simulink model "engine_core"  (R2026a)
settings: Solver=ode23t  StopTime=1039.5715
values from neighbouring files (symbols this model uses):
  Eng = struct()    [AeroDieselEngineParameters.m]
libraries: simulink x2
settings Model: Creator=asus  LastModifiedBy=asus

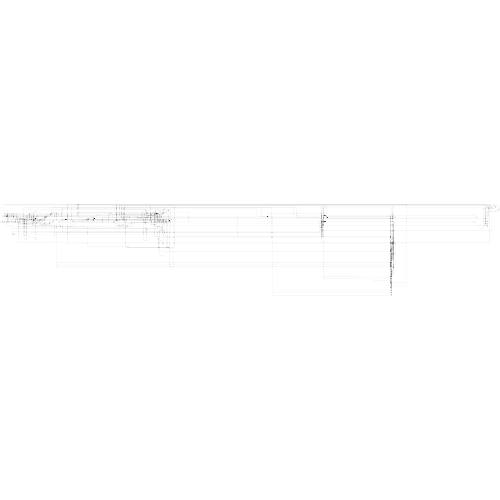
[thumbnail: Simulink's stored preview of the top-level diagram]
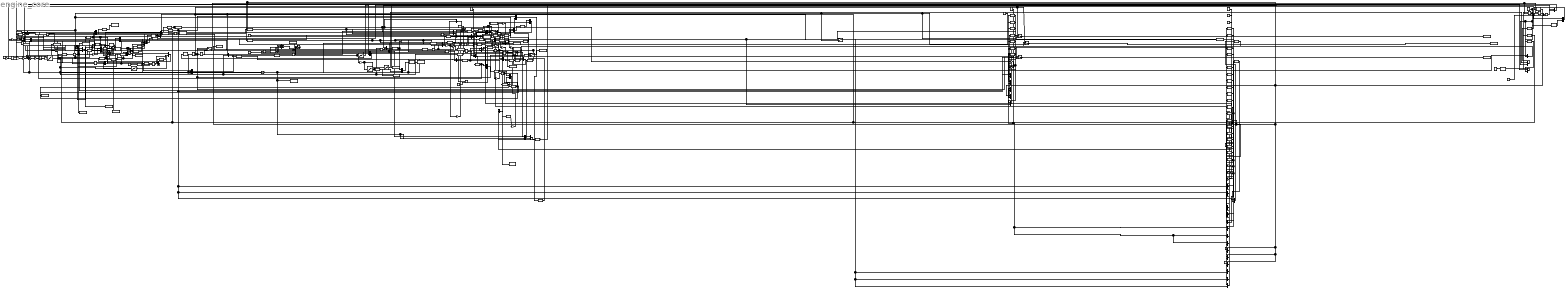
== system engine_core ==
  CmpEngineRunning : simulink/Logic and Bit Operations/Compare To Constant  relop=>  const=400  OutDataTypeStr=boolean
  ConstAlternatorHealth : Constant  Value=Eng.AlternatorHealth_init
  ConstAltitude : FromWorkspace  VariableName=MissionAltitude
  ConstBearingHealth : Constant  Value=Eng.BearingHealth_init
  ConstCoolingHealth : Constant  Value=Eng.CoolingHealth_init
  ConstDropoutNaNVibX : Constant  Value=NaN
  ConstElectricalLoad : Constant  Value=Eng.ElectricalLoad_kW
  ConstEpsilon : Constant  Value=1e-6
  ConstFuelDenomEps : Constant  Value=0.01
  ConstFueldelivHealth : Constant  Value=Eng.FuelDeliveryHealth_init
  ConstInjTimingDeg : Constant  Value=Eng.InjectionTimingDeg_init
  ConstInjhealthC1 : Constant  Value=Eng.InjectorHealth_c1_init
  ConstInjhealthC2 : Constant  Value=Eng.InjectorHealth_c2_init
  ConstInjhealthC3 : Constant  Value=Eng.InjectorHealth_c3_init
  ConstInjhealthC4 : Constant  Value=Eng.InjectorHealth_c4_init
  ConstIsatempoffset : FromWorkspace  VariableName=MissionIsaOffset
  ConstMdotEps : Constant  Value=0.001
  ConstMinrpmFloor : Constant  Value=400
  ConstOilpumpHealth : Constant  Value=Eng.OilPumpHealth_init
  ConstOne : Constant
  ConstPowerfloor : Constant  Value=0.001
  ConstSensorBiasC3 : Constant  Value=Eng.SensorBiasOffset_c3_degC
  ConstTurboEfficiencyDeg : Constant  Value=Eng.TurboEfficiencyDeg_init
  ConstZeroAfr : Constant  Value=0
  ConstZeroFuel : Constant  Value=0
  DivideFuelDeficitRatio : Product  Inputs=*/
  EnvService : ModelReference  ModelNameDialog=environment_service  SimulationMode=Normal  ModelReferenceVersion=1.2
  FcnActualPowerKw : Fcn  Expr=u[1]*(u[2]*2*pi/60)/1000
  FcnAfr : Fcn  Expr=u[1]/u[2]
  FcnAirmdot : Fcn  Expr=0.0017919*(u[1]/2/60)*(u[2]/(287.05*u[3]))
  FcnAlternatorPower : Fcn  Expr=u[1]*u[2]*Eng.AlternatorRatedPower_kW
  FcnBatteryCurrent : Fcn  Expr=u[1]*1000/u[2]
  FcnBatteryNetpower : Fcn  Expr=u[1]-u[2]
  FcnBatteryVoltage : Fcn  Expr=Eng.SystemVoltage_V*(0.85+0.15*u)
  FcnBoostBar : Fcn  Expr=(u[1]-u[2])/1e5
  FcnBsfcPenaltyFactor : Fcn  Expr=1+Eng.TimingDriftBSFCPenalty*u
  FcnCht1Net : Fcn  Expr=u[1]*1000-u[2]
  FcnCht1Reject : Fcn  Expr=Eng.CHTHeatTransferCoeff_W_per_K*(u[1]-u[2])
  FcnCht2Net : Fcn  Expr=u[1]*1000-u[2]
  FcnCht2Reject : Fcn  Expr=Eng.CHTHeatTransferCoeff_W_per_K*(u[1]-u[2])
  FcnCht3Net : Fcn  Expr=u[1]*1000-u[2]
  FcnCht3Reject : Fcn  Expr=Eng.CHTHeatTransferCoeff_W_per_K*(u[1]-u[2])
  FcnCht4Net : Fcn  Expr=u[1]*1000-u[2]
  FcnCht4Reject : Fcn  Expr=Eng.CHTHeatTransferCoeff_W_per_K*(u[1]-u[2])
  FcnEffectiveHeadroom : Fcn  Expr=1+(Eng.TurboAltitudeCompHeadroom-1)*(1-u)
  FcnEgtC1Raw : Fcn  Expr=u[1]+u[2]
  FcnEgtC2Raw : Fcn  Expr=u[1]+u[2]
  FcnEgtC3Raw : Fcn  Expr=u[1]+u[2]
  FcnEgtC4Raw : Fcn  Expr=u[1]+u[2]
  FcnEgtDegc : Fcn  Expr=u[1]+u[2]
  FcnEgtRise : Fcn  Expr=u[1]*1000/(Eng.CpExhaust_J_per_kgK*u[2])
  FcnEgtriseC{1..4} (4 alike) : Fcn  Expr=u[1]*1000/(Eng.CpExhaust_J_per_kgK*u[2])
  FcnExhaustfraction : Fcn  Expr=0.35+0*u[1]+Eng.TimingDriftExhaustPenalty*u[2]
  FcnExhaustmdot : Fcn  Expr=u[1]+u[2]
  FcnExhmdotC{1..4} (4 alike) : Fcn  Expr=u[1]+u[2]
  FcnFrictionScaled : Fcn  Expr=u[1]*(1+Eng.BearingFrictionGain*(1-u[2]))
  FcnFrictionpower : Fcn  Expr=u[1]*(u[2]*2*pi/60)
  FcnFuelFinal : Fcn  Expr=u[1]*u[2]
  FcnFuelFlow : Fcn  Expr=2.0+u[1]*u[2]/1000
  FcnFuelMdotKgs : Fcn  Expr=u/3600
  FcnFuelmdotC{1..4} (4 alike) : Fcn  Expr=u/3600
  FcnFuelpowerKw : Fcn  Expr=u*11.8889
  FcnFuelshareC{1..4} (4 alike) : Fcn  Expr=0.25*u[1]*u[2]
  FcnInjDurationMs : Fcn  Expr=u[1]/u[2]
  FcnInjFlowrate : Fcn  Expr=30*sqrt(u/1500)
  FcnInjQtyMg : Fcn  Expr=(u[1]*1e6/3600)/(4*(u[2]/2/60))
  FcnMapPa : Fcn  Expr=u[1]*u[2]
  FcnMapSealevelRef : Fcn  Expr=101325*u
  FcnMaxDeliverableFuel : Fcn  Expr=Eng.MaxRatedFuelFlow_kg_h*u
  FcnOilHeatTotal : Fcn  Expr=u[1]+u[2]
  FcnOilNet : Fcn  Expr=u[1]-u[2]
  FcnOilReject : Fcn  Expr=Eng.UAOilCooler_W_per_K*(u[1]-u[2])
  FcnOilpressure : Fcn  Expr=u[2]*(Eng.OilPressureIdle_bar+Eng.OilPumpGain_bar_per_rpm*(u[1]-Eng.IdleRPM_crank))
  FcnOilrejectScaled : Fcn  Expr=u[1]*u[2]
  FcnOtherlossesFraction : Fcn  Expr=1-u[1]-Eng.CoolantHeatFraction-u[2]
  FcnPambPa : Fcn  Expr=u*1000
  FcnPrActual : Fcn  Expr=1+u[1]*(u[2]-1)
  FcnPrCompensated : Fcn  Expr=u[1]*u[2]
  FcnPrFinalRef : Fcn  Expr=1+u[1]*(u[2]-1)
  FcnQOtherW : Fcn  Expr=u[1]*u[2]*1000
  FcnQexhaust : Fcn  Expr=u[1]*u[2]
  FcnQexhaustC{1..4} (4 alike) : Fcn  Expr=u[1]*u[2]
  FcnQtotalC{1..4} (4 alike) : Fcn  Expr=u*11.8889
  FcnRadiatorOut : Fcn  Expr=1330*(u[1]-u[2])
  FcnRadiatorScaled : Fcn  Expr=u[1]*u[2]
  FcnRatioNeeded : Fcn  Expr=101325/u
  FcnRefPowerKw : Fcn  Expr=u[1]*(u[2]*2*pi/60)/1000
  FcnRpmFraction : Fcn  Expr=u/Eng.RatedRPM_crank
  FcnRpmRatioSq : Fcn  Expr=(u/Eng.RatedRPM_crank)^2
  FcnTambK : Fcn  Expr=u+273.15
  FcnTcompoutK : Fcn  Expr=u[1]*(1+(u[2]^0.285714-1)/0.7)
  FcnTimingActual : Fcn  Expr=u[1]-Eng.InjectionTimingDriftMax_deg*u[2]
  FcnTintakeDegc : Fcn  Expr=u-273.15
  FcnTintakeK : Fcn  Expr=u[1]-0.75*(u[1]-u[2])
  FcnTorqueFinal : Fcn  Expr=u[1]*u[2]
  FcnTorqueFinal2 : Fcn  Expr=u[1]*u[2]
  FcnTorquePenaltyFactor : Fcn  Expr=1-Eng.TimingDriftTorquePenalty*u
  FcnTorqueScaleFactor : Fcn  Expr=u[1]/u[2]
  FcnTorqueScaledV2 : Fcn  Expr=u[1]*u[2]
  FcnVibrationOrder1x : Fcn  Expr=Eng.VibrationImbalanceGain_g*(1-u[2])*u[1]
  FcnVibrationRmsX : Fcn  Expr=sqrt(Eng.VibrationBaseline_g^2+u^2)
  FcnWorkfraction : Fcn  Expr=u[1]/u[2]
  GainAirmdotPercyl : Gain  Gain=0.25
  GainCht1Rate : Gain  Gain=1/Eng.CHTThermalMass_J_per_K
  GainCht2Rate : Gain  Gain=1/Eng.CHTThermalMass_J_per_K
  GainCht3Rate : Gain  Gain=1/Eng.CHTThermalMass_J_per_K
  GainCht4Rate : Gain  Gain=1/Eng.CHTThermalMass_J_per_K
  GainCoolantRate : Gain  Gain=1/Eng.CoolantThermalMass_J_per_K
  GainFriction : Gain  Gain=Eng.FrictionCoeff_Nm_per_rpm
  GainGearboxReflect : Gain  Gain=1/Eng.GearboxReductionRatio
  GainGearboxToProp : Gain  Gain=1/Eng.GearboxReductionRatio
  GainInvinertia : Gain  Gain=1/Eng.CrankInertia_kgm2
  GainLambda : Gain  Gain=1/Eng.StoichAFR_diesel
  GainLoadfraction : Gain  Gain=1/123.5
  GainMapKpa : Gain  Gain=0.001
  GainOilRate : Gain  Gain=1/Eng.OilThermalMass_J_per_K
  GainProploadcoeff : Gain  Gain=Eng.PropLoadCoeff_Nm_per_prop_rpm2
  GainQcoolant : Gain  Gain=Eng.CoolantHeatFraction
  GainQcoolantDirect : Gain  Gain=1000*(1-Eng.HeadHeatShareOfCoolant)
  GainQhead : Gain  Gain=Eng.HeadHeatShareOfCoolant
  GainQheadC{1..4} (4 alike) : Gain  Gain=Eng.CoolantHeatFraction*Eng.HeadHeatShareOfCoolant
  GainRadstorpm : Gain  Gain=60/(2*pi)
  GainSocRate : Gain  Gain=1000/(Eng.BatteryCapacity_Ah*3600*Eng.SystemVoltage_V)
  GainVibrationRmsZ : Gain  Gain=0.3
  IntChtC{1..4} (4 alike) : Integrator  InitialCondition=Eng.CHTInit_degC
  IntCoolant : Integrator  InitialCondition=Eng.CoolantTempInit_degC
  IntOil : Integrator  InitialCondition=Eng.OilTempInit_degC
  IntSoc : Integrator  InitialCondition=0.8  LimitOutput=on  UpperSaturationLimit=1  LowerSaturationLimit=0
  Integrator : Integrator  InitialCondition=Eng.IdleRPM_crank*2*pi/60
  LutBsfc : Lookup_n-D  NumberOfTableDimensions=1  BreakpointsForDimension1=Eng.BSFCMap.RefPower_kW  Table=Eng.BSFCMap.BSFC_g_per_kWh  ExtrapMethod=Clip  InternalRulePriority=Speed  RndMeth=Simplest
  LutInjTiming : Lookup_n-D  NumberOfTableDimensions=1  BreakpointsForDimension1=Eng.InjectionTimingMap.LoadFraction  Table=Eng.InjectionTimingMap.Timing_degBTDC  ExtrapMethod=Clip  InternalRulePriority=Speed  RndMeth=Simplest
  LutPrFull : Lookup_n-D  NumberOfTableDimensions=1  BreakpointsForDimension1=Eng.TurboBoostMap.RPM_crank  Table=Eng.TurboBoostMap.PressureRatio  ExtrapMethod=Clip  InternalRulePriority=Speed  RndMeth=Simplest
  LutRailPressure : Lookup_n-D  NumberOfTableDimensions=1  BreakpointsForDimension1=Eng.RailPressureMap.LoadFraction  Table=Eng.RailPressureMap.Pressure_bar  ExtrapMethod=Clip  InternalRulePriority=Speed  RndMeth=Simplest
  LutTorquecurve : Lookup_n-D  NumberOfTableDimensions=1  BreakpointsForDimension1=Eng.TorqueCurve.RPM_crank  Table=Eng.TorqueCurve.Torque_Nm  ExtrapMethod=Clip  InternalRulePriority=Speed  RndMeth=Simplest
  MathRpmsquared : Math  Operator=square  SignedPower=on  RndMeth=Zero
  MemoryStuckC3 : Memory
  MinmaxCompfactor : MinMax  Inputs=2
  MinmaxExhmdotFloor : MinMax  Function=max  Inputs=2
  MinmaxFuelActual : MinMax  Inputs=2
  MinmaxFuelDenomFloor : MinMax  Function=max  Inputs=2
  MinmaxFuelmdotFloor : MinMax  Function=max  Inputs=2
  MinmaxFuelpowerFloor : MinMax  Function=max  Inputs=2
  MinmaxRpmFloor : MinMax  Function=max  Inputs=2
  MinmaxRpmfracCap : MinMax  Inputs=2
  MuxActualpwrFuelpwr : Mux  Inputs=2
  MuxAirFuel : Mux  Inputs=2
  MuxAirFuelMdot : Mux  Inputs=2
  MuxBatteryNetpower : Mux  Inputs=2
  MuxCapfracHealth : Mux  Inputs=2
  MuxCht1Coolant : Mux  Inputs=2
  MuxCht1Net : Mux  Inputs=2
  MuxCht2Coolant : Mux  Inputs=2
  MuxCht2Net : Mux  Inputs=2
  MuxCht3Coolant : Mux  Inputs=2
  MuxCht3Net : Mux  Inputs=2
  MuxCht4Coolant : Mux  Inputs=2
  MuxCht4Net : Mux  Inputs=2
  MuxCoolantAmbient : Mux  Inputs=2
  MuxEgtC{1..4} (4 alike) : Mux  Inputs=2
  MuxEgtriseC{1..4} (4 alike) : Mux  Inputs=2
  MuxExhfracTimingdeg : Mux  Inputs=2
  MuxExhmdotC{1..4} (4 alike) : Mux  Inputs=2
  MuxFrictionHealth : Mux  Inputs=2
  MuxFrictionOther : Mux  Inputs=2
  MuxFrictionpower : Mux  Inputs=2
  MuxFuelHealthC{1..4} (4 alike) : Mux  Inputs=2
  MuxFuelTimingpenalty : Mux  Inputs=2
  MuxFuelflowRpm : Mux  Inputs=2
  MuxFuelpowerOtherfrac : Mux  Inputs=2
  MuxFuelpwrExhfrac : Mux  Inputs=2
  MuxImbalance : Mux  Inputs=2
  MuxMapActualRef : Mux  Inputs=2
  MuxMapPambBoost : Mux  Inputs=2
  MuxOilCoolant : Mux  Inputs=2
  MuxOilNet : Mux  Inputs=2
  MuxOilcoolerHealth : Mux  Inputs=2
  MuxOtherlosses : Mux  Inputs=2
  MuxPambPr : Mux  Inputs=2
  MuxPowerVoltage : Mux  Inputs=2
  MuxPrrawCompfactor : Mux  Inputs=2
  MuxQexhC{1..4} (4 alike) : Mux  Inputs=2
  MuxQexhMdot : Mux  Inputs=2
  MuxQtyFlowrate : Mux  Inputs=2
  MuxRadiatorHealth : Mux  Inputs=2
  MuxRefpwrBsfc : Mux  Inputs=2
  MuxRpmMapTintake : Mux  Inputs=3
  MuxRpmOilhealth : Mux  Inputs=2
  MuxTambPr : Mux  Inputs=2
  MuxTcompoutTamb : Mux  Inputs=2
  MuxThrPrfull : Mux  Inputs=2
  MuxThrPrrawRef : Mux  Inputs=2
  MuxTimingDrift : Mux  Inputs=2
  MuxTintakeEgtrise : Mux  Inputs=2
  MuxTorqueFueldeficit : Mux  Inputs=2
  MuxTorqueScale : Mux  Inputs=2
  MuxTorqueTimingpenalty : Mux  Inputs=2
  MuxTrqRpmActualpwr : Mux  Inputs=2
  MuxTrqRpmRefpwr : Mux  Inputs=2
  ProdEnginetorque : Product
  RampSensordriftC3 : simulink/Sources/Ramp  slope=Eng.SensorDriftRate_c3_degC_per_s  start=0  InitialOutput=0
  RandnSensorNoiseC3 : RandomNumber  Variance=Eng.SensorNoiseSigma_c3_degC^2  Seed=42  SampleTime=0.1
  ScopeRpm : Scope
  ScopeTorque : Scope
  StepDropoutOffVibX : Step  Time=Eng.SensorDropoutEndTime_s  SampleTime=0
  StepDropoutOnVibX : Step  Time=Eng.SensorDropoutStartTime_s  SampleTime=0
  StepStuckActiveC3 : Step  Time=Eng.SensorStuckActivationTime_s  SampleTime=0
  StepThrottle : FromWorkspace  VariableName=MissionThrottle
  SumCht3Reported : Sum  Inputs=++++
  SumChtRejects : Sum  Inputs=++++
  SumCoolantHeatin : Sum  Inputs=+++
  SumCoolantNet : Sum  Inputs=+-
  SumDropoutControlVibX : Sum  Inputs=+-
  SumNettorque : Sum  Inputs=+--
  SwitchAfrGate : Switch  Criteria=u2 > Threshold  Threshold=0.5  SaturateOnIntegerOverflow=off  InputSameDT=off
  SwitchDropoutVibX : Switch  Criteria=u2 > Threshold  Threshold=0.5  SaturateOnIntegerOverflow=off  InputSameDT=off
  SwitchEgtC1Gate : Switch  Criteria=u2 > Threshold  Threshold=0.5  SaturateOnIntegerOverflow=off  InputSameDT=off
  SwitchEgtC2Gate : Switch  Criteria=u2 > Threshold  Threshold=0.5  SaturateOnIntegerOverflow=off  InputSameDT=off
  SwitchEgtC3Gate : Switch  Criteria=u2 > Threshold  Threshold=0.5  SaturateOnIntegerOverflow=off  InputSameDT=off
  SwitchEgtC4Gate : Switch  Criteria=u2 > Threshold  Threshold=0.5  SaturateOnIntegerOverflow=off  InputSameDT=off
  SwitchEgtGate : Switch  Criteria=u2 > Threshold  Threshold=0.5  SaturateOnIntegerOverflow=off  InputSameDT=off
  SwitchFuelGate : Switch  Criteria=u2 > Threshold  Threshold=0.5  SaturateOnIntegerOverflow=off  InputSameDT=off
  SwitchStuckC3 : Switch  Criteria=u2 > Threshold  Threshold=0.5  SaturateOnIntegerOverflow=off  InputSameDT=off
  TowsAfr : ToWorkspace  VariableName=afr_out  SaveFormat=Timeseries  SampleTime=-1
  TowsAirmdot : ToWorkspace  VariableName=air_mdot_out  SaveFormat=Timeseries  SampleTime=-1
  TowsAltpower : ToWorkspace  VariableName=alt_power_out  SaveFormat=Timeseries  SampleTime=-1
  TowsAmbientTemp : ToWorkspace  VariableName=ambient_temp_out  SaveFormat=Timeseries  SampleTime=-1
  TowsBattcurrent : ToWorkspace  VariableName=batt_current_out  SaveFormat=Timeseries  SampleTime=-1
  TowsBattvoltage : ToWorkspace  VariableName=batt_voltage_out  SaveFormat=Timeseries  SampleTime=-1
  TowsBoost : ToWorkspace  VariableName=boost_pressure_out  SaveFormat=Timeseries  SampleTime=-1
  TowsCht1 : ToWorkspace  VariableName=cht1_out  SaveFormat=Timeseries  SampleTime=-1
  TowsCht2 : ToWorkspace  VariableName=cht2_out  SaveFormat=Timeseries  SampleTime=-1
  TowsCht3 : ToWorkspace  VariableName=cht3_out  SaveFormat=Timeseries  SampleTime=-1
  TowsCht3Reported : ToWorkspace  VariableName=cht3_reported_out  SaveFormat=Timeseries  SampleTime=-1
  TowsCht4 : ToWorkspace  VariableName=cht4_out  SaveFormat=Timeseries  SampleTime=-1
  TowsCoolant : ToWorkspace  VariableName=coolant_out  SaveFormat=Timeseries  SampleTime=-1
  TowsDensity : ToWorkspace  VariableName=air_density_out  SaveFormat=Timeseries  SampleTime=-1
  TowsEgt : ToWorkspace  VariableName=egt_out  SaveFormat=Timeseries  SampleTime=-1
  TowsEgtC1 : ToWorkspace  VariableName=egt_c1_out  SaveFormat=Timeseries  SampleTime=-1
  TowsEgtC2 : ToWorkspace  VariableName=egt_c2_out  SaveFormat=Timeseries  SampleTime=-1
  TowsEgtC3 : ToWorkspace  VariableName=egt_c3_out  SaveFormat=Timeseries  SampleTime=-1
  TowsEgtC4 : ToWorkspace  VariableName=egt_c4_out  SaveFormat=Timeseries  SampleTime=-1
  TowsFuelflow : ToWorkspace  VariableName=fuel_flow_out  SaveFormat=Timeseries  SampleTime=-1
  TowsInjduration : ToWorkspace  VariableName=inj_duration_out  SaveFormat=Timeseries  SampleTime=-1
  TowsInjqty : ToWorkspace  VariableName=inj_qty_out  SaveFormat=Timeseries  SampleTime=-1
  TowsInjtiming : ToWorkspace  VariableName=inj_timing_out  SaveFormat=Timeseries  SampleTime=-1
  TowsLambda : ToWorkspace  VariableName=lambda_out  SaveFormat=Timeseries  SampleTime=-1
  TowsMap : ToWorkspace  VariableName=map_out  SaveFormat=Timeseries  SampleTime=-1
  TowsOil : ToWorkspace  VariableName=oil_out  SaveFormat=Timeseries  SampleTime=-1
  TowsOilpressure : ToWorkspace  VariableName=oil_pressure_out  SaveFormat=Timeseries  SampleTime=-1
  TowsPressure : ToWorkspace  VariableName=ambient_pressure_out  SaveFormat=Timeseries  SampleTime=-1
  TowsQhead : ToWorkspace  VariableName=q_head_out  SaveFormat=Timeseries  SampleTime=-1
  TowsQtotal : ToWorkspace  VariableName=q_total_out  SaveFormat=Timeseries  SampleTime=-1
  TowsRailpressure : ToWorkspace  VariableName=rail_pressure_out  SaveFormat=Timeseries  SampleTime=-1
  TowsRpm : ToWorkspace  VariableName=rpm_out  SaveFormat=Timeseries  SampleTime=-1
  TowsSoc : ToWorkspace  VariableName=soc_out  SaveFormat=Timeseries  SampleTime=-1
  TowsTintake : ToWorkspace  VariableName=intake_temp_out  SaveFormat=Timeseries  SampleTime=-1
  TowsTorque : ToWorkspace  VariableName=torque_out  SaveFormat=Timeseries  SampleTime=-1
  TowsVibOrder1x : ToWorkspace  VariableName=vib_order1x_out  SaveFormat=Timeseries  SampleTime=-1
  TowsVibRmsX : ToWorkspace  VariableName=vib_rms_x_out  SaveFormat=Timeseries  SampleTime=-1
  TowsVibRmsZ : ToWorkspace  VariableName=vib_rms_z_out  SaveFormat=Timeseries  SampleTime=-1
  wires:
  Integrator/1 -> GainRadstorpm/1
  GainInvinertia/1 -> Integrator/1
  GainGearboxReflect/1 -> SumNettorque/2
  GainGearboxToProp/1 -> MathRpmsquared/1
  GainProploadcoeff/1 -> GainGearboxReflect/1
  MathRpmsquared/1 -> GainProploadcoeff/1
  SumNettorque/1 -> GainInvinertia/1
  FcnTambK/1 -> MuxTcompoutTamb/2, MuxTambPr/1
  MuxPambPr/1 -> FcnMapPa/1
  FcnPrActual/1 -> MuxTambPr/2, MuxPambPr/2
  FcnBoostBar/1 -> TowsBoost/1
  MuxMapPambBoost/1 -> FcnBoostBar/1
  MuxRpmMapTintake/1 -> FcnAirmdot/1
  MuxTorqueScale/1 -> FcnTorqueScaledV2/1
  FcnTorqueScaleFactor/1 -> MuxTorqueScale/2
  MuxMapActualRef/1 -> FcnTorqueScaleFactor/1
  FcnMapSealevelRef/1 -> MuxMapActualRef/2
  FcnPrFinalRef/1 -> FcnMapSealevelRef/1
  MuxThrPrrawRef/1 -> FcnPrFinalRef/1
  FcnPrCompensated/1 -> MuxThrPrfull/2
  FcnMapPa/1 -> MuxMapActualRef/1, MuxRpmMapTintake/2, GainMapKpa/1, MuxMapPambBoost/1
  MuxThrPrfull/1 -> FcnPrActual/1
  MuxTambPr/1 -> FcnTcompoutK/1
  FcnTcompoutK/1 -> MuxTcompoutTamb/1
  MuxTcompoutTamb/1 -> FcnTintakeK/1
  LutBsfc/1 -> MuxRefpwrBsfc/2
  FcnRefPowerKw/1 -> GainLoadfraction/1, MuxRefpwrBsfc/1, LutBsfc/1
  MuxTrqRpmRefpwr/1 -> FcnRefPowerKw/1
  ProdEnginetorque/1 -> MuxTrqRpmRefpwr/1, MuxTorqueScale/1
  FcnInjDurationMs/1 -> TowsInjduration/1
  LutInjTiming/1 -> MuxTimingDrift/1
  GainLoadfraction/1 -> LutRailPressure/1, LutInjTiming/1
  LutRailPressure/1 -> TowsRailpressure/1, FcnInjFlowrate/1
  FcnInjQtyMg/1 -> TowsInjqty/1, MuxQtyFlowrate/1
  FcnInjFlowrate/1 -> MuxQtyFlowrate/2
  MuxQtyFlowrate/1 -> FcnInjDurationMs/1
  FcnTintakeK/1 -> FcnTintakeDegc/1, MuxRpmMapTintake/3
  GainMapKpa/1 -> TowsMap/1
  MinmaxRpmFloor/1 -> MuxFuelflowRpm/2
  ConstMinrpmFloor/1 -> MinmaxRpmFloor/2
  MuxFuelflowRpm/1 -> FcnInjQtyMg/1
  ConstZeroFuel/1 -> SwitchFuelGate/3
  FcnFuelFlow/1 -> SwitchFuelGate/1
  MuxRefpwrBsfc/1 -> FcnFuelFlow/1
  MuxActualpwrFuelpwr/1 -> FcnWorkfraction/1
  MinmaxFuelpowerFloor/1 -> MuxActualpwrFuelpwr/2
  FcnActualPowerKw/1 -> MuxActualpwrFuelpwr/1
  MuxTrqRpmActualpwr/1 -> FcnActualPowerKw/1
  ConstPowerfloor/1 -> MinmaxFuelpowerFloor/2
  ConstMdotEps/1 -> MinmaxExhmdotFloor/2
  SwitchEgtGate/1 -> TowsEgt/1
  MinmaxExhmdotFloor/1 -> MuxQexhMdot/2
  MuxFuelpwrExhfrac/1 -> FcnQexhaust/1
  FcnQexhaust/1 -> MuxQexhMdot/1
  GainOilRate/1 -> IntOil/1
  FcnOilNet/1 -> GainOilRate/1
  GainCoolantRate/1 -> IntCoolant/1
  MuxCht1Coolant/1 -> FcnCht1Reject/1
  FcnCht2Reject/1 -> SumChtRejects/2, MuxCht2Net/2
  GainCht2Rate/1 -> IntChtC2/1
  FcnAirmdot/1 -> GainAirmdotPercyl/1, MuxAirFuel/1, MuxAirFuelMdot/1, TowsAirmdot/1
  SwitchAfrGate/1 -> GainLambda/1, TowsAfr/1
  FcnAfr/1 -> SwitchAfrGate/1
  MuxAirFuel/1 -> FcnAfr/1
  FcnEgtRise/1 -> MuxTintakeEgtrise/2
  MuxQexhMdot/1 -> FcnEgtRise/1
  MuxOilcoolerHealth/1 -> FcnOilrejectScaled/1
  ConstOilpumpHealth/1 -> MuxRpmOilhealth/2, MuxOilcoolerHealth/2
  FcnRadiatorScaled/1 -> SumCoolantNet/2
  MuxRadiatorHealth/1 -> FcnRadiatorScaled/1
  ConstCoolingHealth/1 -> MuxRadiatorHealth/2
  SumCoolantHeatin/1 -> SumCoolantNet/1
  FcnOilReject/1 -> MuxOilcoolerHealth/1
  SumChtRejects/1 -> SumCoolantHeatin/1
  ConstZeroAfr/1 -> SwitchAfrGate/3
  MuxAirFuelMdot/1 -> FcnExhaustmdot/1
  FcnFuelMdotKgs/1 -> MuxAirFuelMdot/2, MinmaxFuelmdotFloor/1
  MuxCht1Net/1 -> FcnCht1Net/1
  FcnCht1Reject/1 -> MuxCht1Net/2, SumChtRejects/1
  MuxCoolantAmbient/1 -> FcnRadiatorOut/1
  FcnRadiatorOut/1 -> MuxRadiatorHealth/1
  SumCoolantNet/1 -> GainCoolantRate/1
  FcnExhaustmdot/1 -> MinmaxExhmdotFloor/1
  ConstEpsilon/1 -> MinmaxFuelmdotFloor/2
  MinmaxFuelmdotFloor/1 -> MuxAirFuel/2
  LutTorquecurve/1 -> ProdEnginetorque/2
  FcnOilpressure/1 -> TowsOilpressure/1
  MuxOilCoolant/1 -> FcnOilReject/1
  MuxRpmOilhealth/1 -> FcnOilpressure/1
  IntChtC2/1 -> TowsCht2/1, MuxCht2Coolant/1
  FcnCht3Net/1 -> GainCht3Rate/1
  MuxCht3Net/1 -> FcnCht3Net/1
  FcnCht3Reject/1 -> MuxCht3Net/2, SumChtRejects/3
  FcnCht2Net/1 -> GainCht2Rate/1
  MuxCht2Net/1 -> FcnCht2Net/1
  MuxCht2Coolant/1 -> FcnCht2Reject/1
  GainCht1Rate/1 -> IntChtC1/1
  FcnCht1Net/1 -> GainCht1Rate/1
  IntOil/1 -> MuxOilCoolant/1, TowsOil/1
  MuxPowerVoltage/1 -> FcnBatteryCurrent/1
  GainSocRate/1 -> IntSoc/1
  FcnBatteryNetpower/1 -> MuxPowerVoltage/1, GainSocRate/1
  MuxBatteryNetpower/1 -> FcnBatteryNetpower/1
  ConstElectricalLoad/1 -> MuxBatteryNetpower/2
  MuxCapfracHealth/1 -> FcnAlternatorPower/1
  ConstAlternatorHealth/1 -> MuxCapfracHealth/2
  MinmaxRpmfracCap/1 -> MuxCapfracHealth/1
  ConstOne/1 -> MinmaxRpmfracCap/2
  FcnRpmFraction/1 -> MinmaxRpmfracCap/1
  MuxCht3Coolant/1 -> FcnCht3Reject/1
  MuxCht4Net/1 -> FcnCht4Net/1
  FcnCht4Net/1 -> GainCht4Rate/1
  GainCht4Rate/1 -> IntChtC4/1
  GainQhead/1 -> TowsQhead/1
  GainQcoolantDirect/1 -> SumCoolantHeatin/3
  GainQcoolant/1 -> GainQcoolantDirect/1, GainQhead/1
  IntChtC1/1 -> MuxCht1Coolant/1, TowsCht1/1
  FcnOilHeatTotal/1 -> MuxOilNet/1
  MuxFrictionOther/1 -> FcnOilHeatTotal/1
  FcnQOtherW/1 -> MuxFrictionOther/2
  MuxOilNet/1 -> FcnOilNet/1
  FcnFrictionpower/1 -> MuxFrictionOther/1
  GainLambda/1 -> TowsLambda/1
  FcnOilrejectScaled/1 -> SumCoolantHeatin/2, MuxOilNet/2
  ConstInjhealthC1/1 -> MuxFuelHealthC1/2
  MuxFuelHealthC1/1 -> FcnFuelshareC1/1
  FcnFuelshareC1/1 -> FcnFuelmdotC1/1, FcnQtotalC1/1
  FcnQtotalC1/1 -> MuxQexhC1/1, GainQheadC1/1
  GainQheadC1/1 -> MuxCht1Net/1
  MuxQexhC1/1 -> FcnQexhaustC1/1
  GainAirmdotPercyl/1 -> MuxExhmdotC4/1, MuxExhmdotC3/1, MuxExhmdotC2/1, MuxExhmdotC1/1
  FcnFuelmdotC1/1 -> MuxExhmdotC1/2
  MuxExhmdotC1/1 -> FcnExhmdotC1/1
  FcnQexhaustC1/1 -> MuxEgtriseC1/1
  FcnExhmdotC1/1 -> MuxEgtriseC1/2
  MuxEgtriseC1/1 -> FcnEgtriseC1/1
  FcnEgtriseC1/1 -> MuxEgtC1/2
  MuxEgtC1/1 -> FcnEgtC1Raw/1
  SwitchEgtC1Gate/1 -> TowsEgtC1/1
  FcnEgtC1Raw/1 -> SwitchEgtC1Gate/1
  ConstInjhealthC2/1 -> MuxFuelHealthC2/2
  MuxFuelHealthC2/1 -> FcnFuelshareC2/1
  FcnFuelshareC2/1 -> FcnQtotalC2/1, FcnFuelmdotC2/1
  FcnQtotalC2/1 -> MuxQexhC2/1, GainQheadC2/1
  GainQheadC2/1 -> MuxCht2Net/1
  MuxQexhC2/1 -> FcnQexhaustC2/1
  FcnFuelmdotC2/1 -> MuxExhmdotC2/2
  MuxExhmdotC2/1 -> FcnExhmdotC2/1
  FcnQexhaustC2/1 -> MuxEgtriseC2/1
  FcnExhmdotC2/1 -> MuxEgtriseC2/2
  MuxEgtriseC2/1 -> FcnEgtriseC2/1
  FcnEgtriseC2/1 -> MuxEgtC2/2
  MuxEgtC2/1 -> FcnEgtC2Raw/1
  ConstInjhealthC3/1 -> MuxFuelHealthC3/2
  MuxFuelHealthC3/1 -> FcnFuelshareC3/1
  FcnFuelshareC3/1 -> FcnQtotalC3/1, FcnFuelmdotC3/1
  FcnQtotalC3/1 -> MuxQexhC3/1, GainQheadC3/1
  GainQheadC3/1 -> MuxCht3Net/1
  MuxQexhC3/1 -> FcnQexhaustC3/1
  FcnFuelmdotC3/1 -> MuxExhmdotC3/2
  MuxExhmdotC3/1 -> FcnExhmdotC3/1
  FcnQexhaustC3/1 -> MuxEgtriseC3/1
  FcnExhmdotC3/1 -> MuxEgtriseC3/2
  MuxEgtriseC3/1 -> FcnEgtriseC3/1
  FcnEgtriseC3/1 -> MuxEgtC3/2
  MuxEgtC3/1 -> FcnEgtC3Raw/1
  ConstInjhealthC4/1 -> MuxFuelHealthC4/2
  MuxFuelHealthC4/1 -> FcnFuelshareC4/1
  FcnFuelshareC4/1 -> FcnQtotalC4/1, FcnFuelmdotC4/1
  FcnQtotalC4/1 -> MuxQexhC4/1, GainQheadC4/1
  GainQheadC4/1 -> MuxCht4Net/1
  MuxQexhC4/1 -> FcnQexhaustC4/1
  FcnFuelmdotC4/1 -> MuxExhmdotC4/2
  MuxExhmdotC4/1 -> FcnExhmdotC4/1
  FcnQexhaustC4/1 -> MuxEgtriseC4/1
  FcnExhmdotC4/1 -> MuxEgtriseC4/2
  SwitchEgtC3Gate/1 -> TowsEgtC3/1
  SwitchEgtC2Gate/1 -> TowsEgtC2/1
  FcnEgtC3Raw/1 -> SwitchEgtC3Gate/1
  FcnEgtC2Raw/1 -> SwitchEgtC2Gate/1
  FcnEffectiveHeadroom/1 -> MinmaxCompfactor/2
  ConstTurboEfficiencyDeg/1 -> FcnEffectiveHeadroom/1
  FcnFuelpowerKw/1 -> MuxFuelpowerOtherfrac/1, MuxFuelpwrExhfrac/1, MinmaxFuelpowerFloor/1, GainQcoolant/1, TowsQtotal/1
  FcnOtherlossesFraction/1 -> MuxFuelpowerOtherfrac/2
  MuxFuelpowerOtherfrac/1 -> FcnQOtherW/1
  IntChtC4/1 -> MuxCht4Coolant/1, TowsCht4/1
  FcnCht4Reject/1 -> SumChtRejects/4, MuxCht4Net/2
  MuxCht4Coolant/1 -> FcnCht4Reject/1
  IntCoolant/1 -> MuxOilCoolant/2, MuxCoolantAmbient/1, MuxCht3Coolant/2, MuxCht4Coolant/2, TowsCoolant/1, MuxCht2Coolant/2, MuxCht1Coolant/2
  FcnAlternatorPower/1 -> TowsAltpower/1, MuxBatteryNetpower/1
  MuxPrrawCompfactor/1 -> FcnPrCompensated/1
  FcnPambPa/1 -> FcnRatioNeeded/1, MuxPambPr/1, MuxMapPambBoost/2
  LutPrFull/1 -> MuxPrrawCompfactor/1, MuxThrPrrawRef/2
  FcnRatioNeeded/1 -> MinmaxCompfactor/1
  MinmaxCompfactor/1 -> MuxPrrawCompfactor/2
  RampSensordriftC3/1 -> SumCht3Reported/2
  IntChtC3/1 -> MuxCht3Coolant/1, TowsCht3/1, SumCht3Reported/1
  GainCht3Rate/1 -> IntChtC3/1
  FcnRpmRatioSq/1 -> MuxImbalance/1
  FcnFrictionScaled/1 -> MuxFrictionpower/1, SumNettorque/3
  MuxFrictionHealth/1 -> FcnFrictionScaled/1
  ConstBearingHealth/1 -> MuxImbalance/2, MuxFrictionHealth/2
  MuxFrictionpower/1 -> FcnFrictionpower/1
  GainRadstorpm/1 -> MuxRpmMapTintake/1, MinmaxRpmFloor/1, FcnRpmFraction/1, MuxTrqRpmActualpwr/2, MuxRpmOilhealth/1, MuxTrqRpmRefpwr/2, CmpEngineRunning/1, LutPrFull/1, GainFriction/1, MuxFrictionpower/2, FcnRpmRatioSq/1, TowsRpm/1, ScopeRpm/1, GainGearboxToProp/1, LutTorquecurve/1
  GainFriction/1 -> MuxFrictionHealth/1
  GainVibrationRmsZ/1 -> TowsVibRmsZ/1
  MuxImbalance/1 -> FcnVibrationOrder1x/1
  EnvService/1 -> FcnPambPa/1, TowsPressure/1
  EnvService/3 -> TowsDensity/1
  EnvService/2 -> SwitchEgtC2Gate/3, FcnTambK/1, SwitchEgtC3Gate/3, SwitchEgtC4Gate/3, SwitchEgtC1Gate/3, SwitchEgtGate/3, MuxCoolantAmbient/2, TowsAmbientTemp/1
  FcnVibrationRmsX/1 -> GainVibrationRmsZ/1, SwitchDropoutVibX/3
  FcnVibrationOrder1x/1 -> FcnVibrationRmsX/1, TowsVibOrder1x/1
  FcnBatteryVoltage/1 -> TowsBattvoltage/1, MuxPowerVoltage/2
  IntSoc/1 -> TowsSoc/1, FcnBatteryVoltage/1
  FcnEgtDegc/1 -> SwitchEgtGate/1
  MuxTintakeEgtrise/1 -> FcnEgtDegc/1
  FcnBatteryCurrent/1 -> TowsBattcurrent/1
  CmpEngineRunning/1 -> SwitchEgtGate/2, SwitchEgtC2Gate/2, SwitchAfrGate/2, SwitchFuelGate/2, SwitchEgtC3Gate/2, SwitchEgtC4Gate/2, SwitchEgtC1Gate/2
  FcnEgtC4Raw/1 -> SwitchEgtC4Gate/1
  SwitchEgtC4Gate/1 -> TowsEgtC4/1
  MuxEgtC4/1 -> FcnEgtC4Raw/1
  FcnEgtriseC4/1 -> MuxEgtC4/2
  MuxEgtriseC4/1 -> FcnEgtriseC4/1
  FcnTintakeDegc/1 -> MuxEgtC3/1, MuxEgtC4/1, MuxEgtC2/1, MuxEgtC1/1, MuxTintakeEgtrise/1, TowsTintake/1
  FcnTorqueFinal/1 -> MuxTorqueTimingpenalty/1
  MuxTimingDrift/1 -> FcnTimingActual/1
  FcnTimingActual/1 -> TowsInjtiming/1
  FcnTorquePenaltyFactor/1 -> MuxTorqueTimingpenalty/2
  MuxTorqueTimingpenalty/1 -> FcnTorqueFinal2/1
  FcnTorqueFinal2/1 -> SumNettorque/1, ScopeTorque/1, TowsTorque/1, MuxTrqRpmActualpwr/1
  MuxExhfracTimingdeg/1 -> FcnExhaustfraction/1
  MuxOtherlosses/1 -> FcnOtherlossesFraction/1
  FcnWorkfraction/1 -> MuxOtherlosses/1, MuxExhfracTimingdeg/1
  FcnExhaustfraction/1 -> MuxQexhC3/2, MuxQexhC4/2, MuxQexhC2/2, MuxQexhC1/2, MuxFuelpwrExhfrac/2, MuxOtherlosses/2
  FcnFuelFinal/1 -> MuxFuelflowRpm/1, FcnFuelpowerKw/1, FcnFuelMdotKgs/1, TowsFuelflow/1, MuxFuelHealthC4/1, MuxFuelHealthC3/1, MuxFuelHealthC2/1, MuxFuelHealthC1/1
  ConstFueldelivHealth/1 -> FcnMaxDeliverableFuel/1
  SwitchFuelGate/1 -> MinmaxFuelActual/2, MinmaxFuelDenomFloor/1
  FcnMaxDeliverableFuel/1 -> MinmaxFuelActual/1
  ConstFuelDenomEps/1 -> MinmaxFuelDenomFloor/2
  FcnBsfcPenaltyFactor/1 -> MuxFuelTimingpenalty/2
  MuxFuelTimingpenalty/1 -> FcnFuelFinal/1
  MinmaxFuelActual/1 -> DivideFuelDeficitRatio/1, MuxFuelTimingpenalty/1
  MinmaxFuelDenomFloor/1 -> DivideFuelDeficitRatio/2
  DivideFuelDeficitRatio/1 -> MuxTorqueFueldeficit/2
  ConstInjTimingDeg/1 -> MuxExhfracTimingdeg/2, MuxTimingDrift/2, FcnBsfcPenaltyFactor/1, FcnTorquePenaltyFactor/1
  MuxTorqueFueldeficit/1 -> FcnTorqueFinal/1
  FcnTorqueScaledV2/1 -> MuxTorqueFueldeficit/1
  ConstSensorBiasC3/1 -> SumCht3Reported/3
  RandnSensorNoiseC3/1 -> SumCht3Reported/4
  SumCht3Reported/1 -> SwitchStuckC3/3
  StepStuckActiveC3/1 -> SwitchStuckC3/2
  MemoryStuckC3/1 -> SwitchStuckC3/1
  SwitchStuckC3/1 -> MemoryStuckC3/1, TowsCht3Reported/1
  ConstDropoutNaNVibX/1 -> SwitchDropoutVibX/1
  StepDropoutOnVibX/1 -> SumDropoutControlVibX/1
  StepDropoutOffVibX/1 -> SumDropoutControlVibX/2
  SumDropoutControlVibX/1 -> SwitchDropoutVibX/2
  SwitchDropoutVibX/1 -> TowsVibRmsX/1
  ConstAltitude/1 -> EnvService/1
  ConstIsatempoffset/1 -> EnvService/2
  StepThrottle/1 -> MuxThrPrrawRef/1, MuxThrPrfull/1, ProdEnginetorque/1
